simulink model "MRAC_sim"  (R2020b)
settings: Solver=VariableStepAuto  StartTime=0.0  StopTime=10.0  RelTol=1e-3
settings Model: Creator=surya  LastModifiedBy=surya

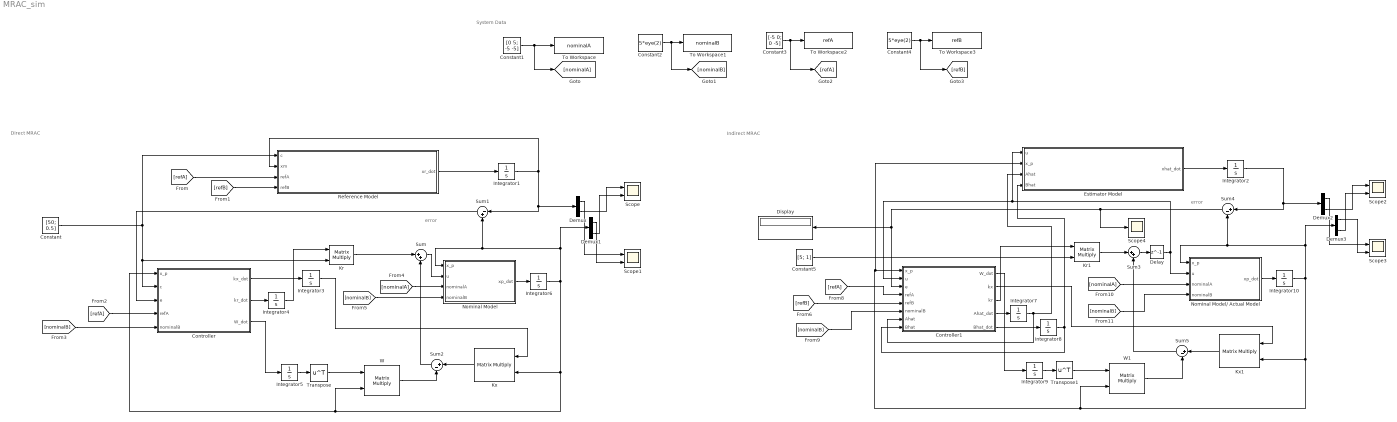
== system MRAC_sim ==
  note: Indirect MRAC
  note: error
  note: System Data
  note: Direct MRAC
  note: error
  Constant : Constant  Value=[50; 0.5]
  Constant1 : Constant  Value=[0 5; -5 -5]
  Constant2 : Constant  Value=5*eye(2)
  Constant3 : Constant  Value=[-5 0; 0 -5]
  Constant4 : Constant  Value=5*eye(2)
  Constant5 : Constant  Value=[5; 1]
  Controller : MATLAB Function  TreatAsAtomicUnit=on
  Controller1 : MATLAB Function  TreatAsAtomicUnit=on
  Delay : Delay  DelayLength=1  InitialCondition=[0;0]
  Demux{,1..3} (4 alike) : Demux  Outputs=2
  Display : Display
  Estimator Model : MATLAB Function  TreatAsAtomicUnit=on
  Integrator{1..2,6,10} (4 alike) : Integrator  InitialCondition=[0; 0]
  Integrator3 : Integrator
  Integrator4 : Integrator  InitialCondition=eye(2)
  Integrator5 : Integrator
  Integrator7 : Integrator  InitialCondition=[-5 0; 0 -5]
  Integrator8 : Integrator  InitialCondition=5*eye(2)
  Integrator9 : Integrator  InitialCondition=zeros([2,2])
  Kr : Product  Multiplication=Matrix(*)
  Kr1 : Product  Multiplication=Matrix(*)
  Kx : Product  Multiplication=Matrix(*)
  Kx1 : Product  Multiplication=Matrix(*)
  Nominal Model : MATLAB Function  TreatAsAtomicUnit=on
  Nominal Model/ Actual Model : MATLAB Function  TreatAsAtomicUnit=on
  Reference Model : MATLAB Function  TreatAsAtomicUnit=on
  Scope{,1..3} (4 alike) : Scope  NumInputPorts=2
  Scope4 : Scope
  Sum : Sum  Inputs=|++
  Sum1 : Sum  Inputs=|-+
  Sum2 : Sum  Inputs=|+-
  Sum3 : Sum  Inputs=|++
  Sum4 : Sum  Inputs=|+-
  Sum5 : Sum  Inputs=|+-
  To Workspace : ToWorkspace  VariableName=nominalA  SaveFormat=Timeseries  SampleTime=-1
  To Workspace1 : ToWorkspace  VariableName=nominalB  SaveFormat=Timeseries  SampleTime=-1
  To Workspace2 : ToWorkspace  VariableName=refA  SaveFormat=Timeseries  SampleTime=-1
  To Workspace3 : ToWorkspace  VariableName=refB  SaveFormat=Timeseries  SampleTime=-1
  Transpose : Math  Operator=transpose  SaturateOnIntegerOverflow=on
  Transpose1 : Math  Operator=transpose  SaturateOnIntegerOverflow=on
  W : Product  Multiplication=Matrix(*)
  W1 : Product  Multiplication=Matrix(*)
  wires:
  Reference Model/1(xr_dot) -> Integrator1/1
  Integrator1/1 -> Reference Model/2(xm), Demux/1, Sum1/1
  Kr/1 -> Sum/1
  Constant/1 -> Controller/2(c), Kr/2, Reference Model/1(c)
  Constant1/1 -> [nominalA], To Workspace/1
  Constant2/1 -> [nominalB], To Workspace1/1
  Constant3/1 -> [refA], To Workspace2/1
  Integrator6/1 -> Demux1/1, Sum1/2, Nominal Model/1(x_p), Controller/1(x_p), W/2, Kx/2
  Sum1/1 -> Controller/3(e)
  Controller/1(kx_dot) -> Integrator3/1
  Controller/2(kr_dot) -> Integrator4/1
  Controller/3(W_dot) -> Integrator5/1
  Integrator3/1 -> Kx/1
  Integrator4/1 -> Kr/1
  Kx/1 -> Sum2/1
  Sum2/1 -> Sum/2
  Sum/1 -> Nominal Model/2(u)
  Nominal Model/1(xp_dot) -> Integrator6/1
  W/1 -> Sum2/2
  Constant4/1 -> [refB], To Workspace3/1
  [refA] -> Reference Model/3(refA)
  [refB] -> Reference Model/4(refB)
  [nominalB] -> Controller/5(nominalB)
  [refA] -> Controller/4(refA)
  [nominalB] -> Nominal Model/4(nominalB)
  [nominalA] -> Nominal Model/3(nominalA)
  Integrator5/1 -> Transpose/1
  Transpose/1 -> W/1
  Demux/1 -> Scope1/1
  Demux1/1 -> Scope1/2
  Demux1/2 -> Scope/2
  Demux/2 -> Scope/1
  Kr1/1 -> Sum3/1
  Sum5/1 -> Sum3/2
  Kx1/1 -> Sum5/1
  Controller1/5(Bhat_dot) -> Integrator8/1
  Controller1/4(Ahat_dot) -> Integrator7/1
  Integrator2/1 -> Demux2/1, Sum4/1
  Constant5/1 -> Kr1/2
  Demux3/2 -> Scope2/2
  Demux3/1 -> Scope3/2
  [refA] -> Controller1/4(refA)
  [nominalB] -> Nominal Model/ Actual Model/4(nominalB)
  Controller1/1(W_dot) -> Integrator9/1
  Sum4/1 -> Scope4/1, Controller1/3(e), Display/1
  Integrator9/1 -> Transpose1/1
  Transpose1/1 -> W1/1
  Estimator Model/1(xhat_dot) -> Integrator2/1
  Integrator7/1 -> Controller1/7(Ahat), Estimator Model/3(Ahat)
  Demux2/1 -> Scope3/1
  Integrator10/1 -> Demux3/1, Sum4/2, Nominal Model/ Actual Model/1(x_p), Estimator Model/2(x_p), Controller1/1(x_p), W1/2, Kx1/2
  [nominalA] -> Nominal Model/ Actual Model/3(nominalA)
  Demux2/2 -> Scope2/1
  W1/1 -> Sum5/2
  Integrator8/1 -> Controller1/8(Bhat), Estimator Model/4(Bhat)
  [nominalB] -> Controller1/6(nominalB)
  Nominal Model/ Actual Model/1(xp_dot) -> Integrator10/1
  Controller1/3(kr) -> Kr1/1
  Controller1/2(kx) -> Kx1/1
  [refB] -> Controller1/5(refB)
  Sum3/1 -> Delay/1
  Delay/1 -> Controller1/2(u), Estimator Model/1(u), Nominal Model/ Actual Model/2(u)

== matlab function MRAC_sim/Reference Model ==
  data: c input; xm input; xr_dot output; refA input; refB input
function xr_dot = fcn(c, xm, refA, refB)

xr_dot = refA*xm + refB*c;

== matlab function MRAC_sim/Controller1 ==
  data: W_dot output; kx output; kr output; Ahat_dot output; x_p input; u input; e input; Bhat_dot output; refA input; refB input; nominalB input; Ahat input; Bhat input
function [W_dot, kx, kr, Ahat_dot, Bhat_dot] = fcn(x_p, u, e, refA, refB, nominalB, Ahat, Bhat)

gamma_a = 0;
gamma_b = 0;
gamma_w = 2;
%P = calc_P(refA, eye(2));
P = [0.1 0; 0 0.1];

Ahat_dot = gamma_a*x_p*e'*P;
Bhat_dot = gamma_b*u*e'*P;
W_dot = gamma_w*x_p*e'*P*nominalB;

if Bhat ~= [0 0; 0 0]
    kx = -inv(Bhat)*(Ahat - refA);
    kr = inv(Bhat)*refB;
else
    kx = zeros([length(x_p),length(x_p)]);
    kr = 0.001*eye(length(u));

end

== matlab function MRAC_sim/Controller ==
  data: kx_dot output; x_p input; c input; e input; kr_dot output; W_dot output; refA input; nominalB input
function [kx_dot, kr_dot, W_dot] = fcn(x_p, c, e, refA, nominalB)

gamma_x = 250;
gamma_r = 30;
gamma_w = 2300;
%P = calc_P(refA, eye(2));
P = [0.1 0; 0 0.1];

kx_dot = gamma_x*x_p*e'*P*nominalB;
kr_dot = gamma_r*c*e'*P*nominalB;
W_dot = gamma_w*x_p*e'*P*nominalB;

end

== matlab function MRAC_sim/Nominal Model ==
  data: xp_dot output; x_p input; u input; nominalA input; nominalB input
function xp_dot  = fcn(x_p, u, nominalA, nominalB)

xp_dot = nominalA*x_p + nominalB*u;

end

== matlab function MRAC_sim/Nominal Model// Actual Model ==
  data: xp_dot output; x_p input; u input; nominalA input; nominalB input
function xp_dot  = fcn(x_p, u, nominalA, nominalB)

xp_dot = nominalA*x_p + nominalB*u;

end

== matlab function MRAC_sim/Estimator Model ==
  data: u input; x_p input; xhat_dot output size=2; Ahat input; Bhat input
function xhat_dot = fcn(u, x_p, Ahat, Bhat)

xhat_dot = Ahat*x_p + Bhat*u;

end
